simulink model "flightControlSystem"  (R2024b)
settings: Solver=ode3  StartTime=0  StopTime=TFinal  FixedStep=Ts  RelTol=1e-3  EnableMultiTasking=on
undefined symbols (not defined in the file): codertarget, Controller, DiscIntNeverNeededParam, Discrete, Estimator, g, gray, init, Sensors, Time, Ts, var_acc_angle_N, var_bias_gyr_N, var_gyro_p_N, Vehicle
libraries: simulink x37, slpidlib x4, ctrlSharedLib x4, simulink_extras x3, sharedtransform x3, vrlib x2, parrotlib x1
(part 3 of 3)

== system flightControlSystem/Control System/State Estimator/XY Position Estimator/EstimatorVelocity/Angular velocity compensation for optical flow ==
  note: Optical flow readings are affected by both linear and angular velocity of the drone. We need to subtract the effect of angular velocity before using the flow data
  z_estimate : Inport
  Angular velocity w/o bias : Inport  Port=2
  Abs : Abs  SaturateOnIntegerOverflow=off
  Data Type Conversion : DataTypeConversion  SaturateOnIntegerOverflow=off  RndMeth=Floor
  Demux : Demux  Outputs=2
  Gain1 : Gain  Gain=-1
  Mux : Mux  Inputs=2
  Selector : Selector  InputPortWidth=3  IndexOptions=Index vector (dialog)  Indices=[1 2]  OutputSizes=1
  prod : Product  Inputs=**
  angular velocity correction : Outport
  wires:
  Gain1/1 -> Mux/1
  Mux/1 -> Data Type Conversion/1
  Demux/2 -> Gain1/1
  Data Type Conversion/1 -> angular velocity correction/1
  prod/1 -> Demux/1
  z_estimate/1 -> Abs/1
  Demux/1 -> Mux/2
  Selector/1 -> prod/2
  Abs/1 -> prod/1
  Angular velocity w/o bias/1 -> Selector/1

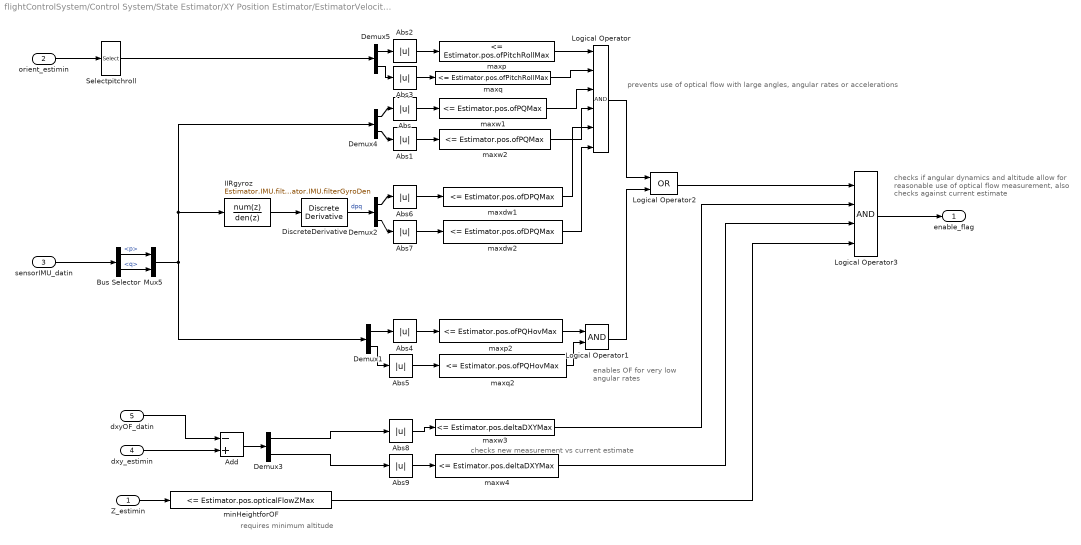
== system flightControlSystem/Control System/State Estimator/XY Position Estimator/EstimatorVelocity/DataHandling ==
  note: prevents use of optical flow with large angles, angular rates or accelerations
  note: enables OF for very
      | low angular rates
  note: checks if angular dynamics and altitude allow for
      | reasonable use of optical flow measurement,
      | also checks against current estimate
  note: checks new measurement vs current estimate
  note: requires minimum altitude
  Z_estimin : Inport
  orient_estimin : Inport  Port=2
  sensorIMU_datin : Inport  Port=3
  dxy_estimin : Inport  Port=4
  dxyOF_datin : Inport  Port=5
  Abs{,1..9} (10 alike) : Abs  SaturateOnIntegerOverflow=off
  Add : Sum  Inputs=-+
  Bus Selector : BusSelector  OutputSignals=p,q
  Demux{1..5} (5 alike) : Demux  Outputs=2
  DiscreteDerivative : simulink/Discrete/Discrete Derivative  gainval=1.0  ICPrevScaledInput=0.0  OutMin=[]  OutMax=[]  OutDataType=fixdt(1, 16)  OutScaling=2^-10  DoSatur=off
  IIRgyroz : DiscreteFilter  Numerator=Estimator.IMU.filterGyroNum  Denominator=Estimator.IMU.filterGyroDen
  Logical Operator : Logic  Inputs=6  AllPortsSameDT=off  OutDataTypeStr=boolean
  Logical Operator1 : Logic  AllPortsSameDT=off  OutDataTypeStr=boolean
  Logical Operator2 : Logic  Operator=OR  AllPortsSameDT=off  OutDataTypeStr=boolean
  Logical Operator3 : Logic  Inputs=4  AllPortsSameDT=off  OutDataTypeStr=boolean
  Mux5 : Mux  Inputs=2
  Selectpitchroll : Selector  InputPortWidth=3  IndexOptions=Index vector (dialog)  Indices=[2 3]  OutputSizes=1
  maxdw1 : simulink/Logic and Bit Operations/Compare To Constant  relop=<=  const=Estimator.pos.ofDPQMax  OutDataTypeStr=boolean
  maxdw2 : simulink/Logic and Bit Operations/Compare To Constant  relop=<=  const=Estimator.pos.ofDPQMax  OutDataTypeStr=boolean
  maxp : simulink/Logic and Bit Operations/Compare To Constant  relop=<=  const=Estimator.pos.ofPitchRollMax  OutDataTypeStr=boolean
  maxp2 : simulink/Logic and Bit Operations/Compare To Constant  relop=<=  const=Estimator.pos.ofPQHovMax  OutDataTypeStr=boolean
  maxq : simulink/Logic and Bit Operations/Compare To Constant  relop=<=  const=Estimator.pos.ofPitchRollMax  OutDataTypeStr=boolean
  maxq2 : simulink/Logic and Bit Operations/Compare To Constant  relop=<=  const=Estimator.pos.ofPQHovMax  OutDataTypeStr=boolean
  maxw1 : simulink/Logic and Bit Operations/Compare To Constant  relop=<=  const=Estimator.pos.ofPQMax  OutDataTypeStr=boolean
  maxw2 : simulink/Logic and Bit Operations/Compare To Constant  relop=<=  const=Estimator.pos.ofPQMax  OutDataTypeStr=boolean
  maxw3 : simulink/Logic and Bit Operations/Compare To Constant  relop=<=  const=Estimator.pos.deltaDXYMax  OutDataTypeStr=boolean
  maxw4 : simulink/Logic and Bit Operations/Compare To Constant  relop=<=  const=Estimator.pos.deltaDXYMax  OutDataTypeStr=boolean
  minHeightforOF : simulink/Logic and Bit Operations/Compare To Constant  relop=<=  const=Estimator.pos.opticalFlowZMax  OutDataTypeStr=boolean
  enable_flag : Outport  VectorParamsAs1DForOutWhenUnconnected=off
  wires:
  minHeightforOF/1 -> Logical Operator3/4
  IIRgyroz/1 -> DiscreteDerivative/1
  Mux5/1 -> Demux1/1, Demux4/1, IIRgyroz/1
  maxw4/1 -> Logical Operator3/3
  maxw3/1 -> Logical Operator3/2
  dxyOF_datin/1 -> Add/1
  Demux3/2 -> Abs9/1
  Demux3/1 -> Abs8/1
  dxy_estimin/1 -> Add/2
  Add/1 -> Demux3/1
  Abs9/1 -> maxw4/1
  Abs8/1 -> maxw3/1
  Logical Operator2/1 -> Logical Operator3/1
  Logical Operator3/1 -> enable_flag/1
  DiscreteDerivative/1 -> Demux2/1  "dpq"
  Demux2/2 -> Abs7/1
  Demux2/1 -> Abs6/1
  Abs7/1 -> maxdw2/1
  Abs6/1 -> maxdw1/1
  Logical Operator1/1 -> Logical Operator2/2
  Demux1/2 -> Abs5/1
  Demux1/1 -> Abs4/1
  Abs5/1 -> maxq2/1
  Abs4/1 -> maxp2/1
  Abs3/1 -> maxq/1
  Abs2/1 -> maxp/1
  Demux4/2 -> Abs1/1
  Demux4/1 -> Abs/1
  Abs1/1 -> maxw2/1
  Abs/1 -> maxw1/1
  Z_estimin/1 -> minHeightforOF/1
  Logical Operator/1 -> Logical Operator2/1
  maxw1/1 -> Logical Operator/3
  Bus Selector/1 -> Mux5/1  "<p>"
  Selectpitchroll/1 -> Demux5/1
  sensorIMU_datin/1 -> Bus Selector/1
  maxq2/1 -> Logical Operator1/2
  Bus Selector/2 -> Mux5/2  "<q>"
  maxp/1 -> Logical Operator/1
  maxw2/1 -> Logical Operator/4
  orient_estimin/1 -> Selectpitchroll/1
  maxdw1/1 -> Logical Operator/5
  maxdw2/1 -> Logical Operator/6
  maxq/1 -> Logical Operator/2
  Demux5/1 -> Abs2/1
  Demux5/2 -> Abs3/1
  maxp2/1 -> Logical Operator1/1

== system flightControlSystem/Control System/State Estimator/XY Position Estimator/EstimatorVelocity/xy velocity w//o angular velocity compensation ==
  note: Optical flow raw readings are converted to velocity in m/s based on the estimated altitude
  optical_flow : Inport
  z_estimate : Inport  Port=2
  " " : Product  Inputs=**
  Compare To Constant : simulink/Logic and Bit Operations/Compare To Constant  relop=<  const=200*4  OutDataTypeStr=boolean
  Counter Free-Running : simulink/Sources/Counter Free-Running  NumBits=32  tsamp=-1
  Gain : Gain  Gain=-1
  Select dxy : Selector  InputPortWidth=3  IndexOptions=Index vector (dialog)  Indices=[1 2]  OutputSizes=1
  Switch : Switch  Criteria=u2 > Threshold  SaturateOnIntegerOverflow=off  InputSameDT=off
  opticalFlowErrorCorrect : Gain  Gain=1.15
  optical_flow_dx_dy : Outport
  wires:
  Select dxy/1 -> optical_flow_dx_dy/1  "optical_flow_dx_dy"
  " "/1 -> opticalFlowErrorCorrect/1
  opticalFlowErrorCorrect/1 -> Switch/3
  Gain/1 -> " "/2
  Switch/1 -> Select dxy/1
  Counter Free-Running/1 -> Compare To Constant/1
  Compare To Constant/1 -> Switch/2
  optical_flow/1 -> " "/1, Switch/1
  z_estimate/1 -> Gain/1

== matlab function flightControlSystem/Image Processing System/Deviation Measurement/MATLAB Function2 ==
  data: err input; iae output; valid input; Ts input; reset input
function iae = metricIAE(err, valid, Ts, reset)
% metricIAE
% Discrete Integral of Absolute Error

persistent acc
if isempty(acc)
    acc = single(0);
end

if reset
    acc = single(0);
else
    if valid ~= 0
        acc = acc + abs(single(err)) * single(Ts);
    end
end

iae = acc;
end

== matlab function flightControlSystem/Image Processing System/Deviation Measurement/MATLAB Function3 ==
  data: err input; itae output; valid input; Ts input; reset input
function itae = metricITAE(err, valid, Ts, reset)
% metricITAE
% Discrete Integral of Time-weighted Absolute Error

persistent acc tNow
if isempty(acc)
    acc  = single(0);
    tNow = single(0);
end

if reset
    acc  = single(0);
    tNow = single(0);
else
    if valid ~= 0
        acc = acc + tNow * abs(single(err)) * single(Ts);
    end
    tNow = tNow + single(Ts);
end

itae = acc;
end

== matlab function flightControlSystem/Image Processing System/Deviation Measurement/MATLAB Function4 ==
  data: R input; G input; B input; d_cm output; e_px output; cm_per_px output; trackW_px output; valid output; offTrack output; IAE output; ITAE output; MAE output; maxErr output; offTime output; offRatio output; validRatio output; debugImg output; headingVec input
function [d_cm, e_px, cm_per_px, trackW_px, valid, offTrack, ...
          IAE, ITAE, MAE, maxErr, offTime, offRatio, validRatio, ...
          debugImg] = fcn(R, G, B, headingVec)

%#codegen

% ============================================================
% PARAMETERS
% ============================================================
rows       = int32(120);
cols       = int32(160);

centerRow  = single(60);
centerCol  = single(80);

redThr     = single(200);   % red detection threshold
trackW_cm  = single(10);    % real track width [cm]
thr_cm     = single(10);    % off-track threshold [cm]
Ts         = single(0.2);   % actual execution sample time of this block

% Cross-section settings
normalHalf     = int32(35);   % half-length of each cross-section [px]
minRunLen      = int32(3);    % minimum contiguous red samples in a section
numSections    = int32(9);    % number of cross-sections along heading

% Section offsets along heading [px]
secOffsets = int32([-12 -9 -6 -3 0 3 6 9 12]);

% ============================================================
% PERSISTENT STATES
% ============================================================
persistent last_d_cm last_e_px last_cm_per_px last_trackW_px
persistent IAE_acc ITAE_acc MAE_sum MAE_count maxErr_val
persistent offTime_acc offCount totalCount validCount tNow
persistent last_trackPtR last_trackPtC
persistent last_hR last_hC
persistent last_dirR last_dirC

if isempty(last_d_cm)
    last_d_cm       = single(0);
    last_e_px       = single(0);
    last_cm_per_px  = single(0);
    last_trackW_px  = single(1);

    IAE_acc         = single(0);
    ITAE_acc        = single(0);
    MAE_sum         = single(0);
    MAE_count       = single(0);
    maxErr_val      = single(0);

    offTime_acc     = single(0);
    offCount        = single(0);
    totalCount      = single(0);
    validCount      = single(0);
    tNow            = single(0);

    last_trackPtR   = centerRow;
    last_trackPtC   = centerCol;

    % Default heading = upward in image plane
    last_hR         = single(-1);
    last_hC         = single(0);

    % Default fitted direction
    last_dirR       = single(-1);
    last_dirC       = single(0);
end

% ============================================================
% HEADING NORMALIZATION
% headingVec is interpreted in image coordinates [row, col]
% ============================================================
hR = single(headingVec(1));
hC = single(headingVec(2));

hNorm = sqrt(hR*hR + hC*hC);

if hNorm > single(1e-6)
    hR = hR / hNorm;
    hC = hC / hNorm;
    last_hR = hR;
    last_hC = hC;
else
    hR = last_hR;
    hC = last_hC;
end

% Normal to heading in image plane
nR = -hC;
nC =  hR;

% ============================================================
% DEBUG IMAGE INIT
% ============================================================
debugImg = zeros(rows, cols, 3, 'uint8');
debugImg(:,:,1) = uint8(R);
debugImg(:,:,2) = uint8(G);
debugImg(:,:,3) = uint8(B);

% ============================================================
% STORAGE FOR VALID CROSS-SECTIONS
% ============================================================
secValid   = false(1, numSections);
secCenterT = zeros(1, numSections, 'single');  % lateral center along normal
secWidth   = zeros(1, numSections, 'single');  % width in px along normal
secPtR     = zeros(1, numSections, 'single');  % detected center point row
secPtC     = zeros(1, numSections, 'single');  % detected center point col
secWeight  = zeros(1, numSections, 'single');

% ============================================================
% SCAN MULTIPLE CROSS-SECTIONS ORTHOGONAL TO HEADING
% ============================================================
for i = 1:numSections
    s = single(secOffsets(i));  % offset along heading from image center

    % Base point of the current cross-section
    baseR = centerRow + s * hR;
    baseC = centerCol + s * hC;

    % Search along normal direction
    currStart = int32(0);
    currLen   = int32(0);
    bestStart = int32(0);
    bestEnd   = int32(-1);
    bestLen   = int32(0);

    prevIsRed = false;

    for t = -normalHalf:normalHalf
        rr = int32(round(baseR + single(t) * nR));
        cc = int32(round(baseC + single(t) * nC));

        isRed = false;

        if rr >= 1 && rr <= rows && cc >= 1 && cc <= cols
            Rv = single(R(rr, cc));
            Gv = single(G(rr, cc));
            Bv = single(B(rr, cc));

            isRed = (Rv - single(0.5)*Gv - single(0.5)*Bv) > redThr;
        end

        if isRed
            if ~prevIsRed
                currStart = t;
                currLen   = int32(1);
            else
                currLen = currLen + int32(1);
            end
        else
            if prevIsRed
                if currLen > bestLen
                    bestLen   = currLen;
                    bestStart = currStart;
                    bestEnd   = t - int32(1);
                end
            end
            currLen = int32(0);
        end

        prevIsRed = isRed;
    end

    % Handle run reaching the end
    if prevIsRed
        if currLen > bestLen
            bestLen   = currLen;
            bestStart = currStart;
            bestEnd   = normalHalf;
        end
    end

    % Accept only meaningful runs
    if bestLen >= minRunLen
        centerT = single(bestStart + bestEnd) * single(0.5);
        widthPx = single(bestEnd - bestStart + int32(1));

        ptR = baseR + centerT * nR;
        ptC = baseC + centerT * nC;

        secValid(i)   = true;
        secCenterT(i) = centerT;
        secWidth(i)   = widthPx;
        secPtR(i)     = ptR;
        secPtC(i)     = ptC;

        % Weight:
        % wider run = more confidence
        % closer to center = slightly more weight
        secWeight(i) = widthPx / (single(1) + single(0.08) * abs(s));
    end
end

% ============================================================
% AGGREGATE CROSS-SECTIONS
% ============================================================
sumW      = single(0);
sumT      = single(0);
sumWidth  = single(0);
sumPtR    = single(0);
sumPtC    = single(0);
numValid  = int32(0);

for i = 1:numSections
    if secValid(i)
        w = secWeight(i);

        sumW     = sumW + w;
        sumT     = sumT + w * secCenterT(i);
        sumWidth = sumWidth + w * secWidth(i);
        sumPtR   = sumPtR + w * secPtR(i);
        sumPtC   = sumPtC + w * secPtC(i);
        numValid = numValid + int32(1);
    end
end

if numValid > 0 && sumW > single(1e-6)
    e = sumT / sumW;            % signed lateral error in pixels along normal
    w_px = sumWidth / sumW;     % estimated track width in pixels
    trackPtR = sumPtR / sumW;   % estimated local centerline point
    trackPtC = sumPtC / sumW;

    if w_px < single(1)
        w_px = single(1);
    end

    cmpp = trackW_cm / w_px;
    d = e * cmpp;

    d_cm       = d;
    e_px       = e;
    cm_per_px  = cmpp;
    trackW_px  = w_px;
    valid      = uint8(1);

    last_d_cm      = d_cm;
    last_e_px      = e_px;
    last_cm_per_px = cm_per_px;
    last_trackW_px = trackW_px;

    last_trackPtR  = trackPtR;
    last_trackPtC  = trackPtC;
else
    d_cm       = last_d_cm;
    e_px       = last_e_px;
    cm_per_px  = last_cm_per_px;
    trackW_px  = last_trackW_px;
    valid      = uint8(0);

    trackPtR   = last_trackPtR;
    trackPtC   = last_trackPtC;
end

% ============================================================
% FIT LOCAL CENTERLINE FROM THE YELLOW POINTS
% weighted line fit / principal direction
% ============================================================
if numValid >= int32(2) && sumW > single(1e-6)
    meanR = sumPtR / sumW;
    meanC = sumPtC / sumW;

    Srr = single(0);
    Scc = single(0);
    Src = single(0);

    for i = 1:numSections
        if secValid(i)
            dr = secPtR(i) - meanR;
            dc = secPtC(i) - meanC;
            w  = secWeight(i);

            Srr = Srr + w * dr * dr;
            Scc = Scc + w * dc * dc;
            Src = Src + w * dr * dc;
        end
    end

    theta = single(0.5) * atan2(single(2) * Src, Srr - Scc);

    dirR = cos(theta);
    dirC = sin(theta);

    dirNorm = sqrt(dirR*dirR + dirC*dirC);
    if dirNorm > single(1e-6)
        dirR = dirR / dirNorm;
        dirC = dirC / dirNorm;

        % Keep orientation roughly aligned with heading to avoid sign flips
        if dirR*hR + dirC*hC < single(0)
            dirR = -dirR;
            dirC = -dirC;
        end

        last_dirR = dirR;
        last_dirC = dirC;
    else
        dirR = last_dirR;
        dirC = last_dirC;
    end
else
    dirR = last_dirR;
    dirC = last_dirC;
end

% ============================================================
% OFF TRACK
% ============================================================
if valid ~= 0
    offTrack = uint8(abs(d_cm) > thr_cm);
else
    offTrack = uint8(0);
end

% ============================================================
% METRICS
% ============================================================
totalCount = totalCount + single(1);

if valid ~= 0
    errAbs = abs(d_cm);

    IAE_acc   = IAE_acc  + errAbs * Ts;
    ITAE_acc  = ITAE_acc + tNow * errAbs * Ts;

    MAE_sum   = MAE_sum + errAbs;
    MAE_count = MAE_count + single(1);

    if errAbs > maxErr_val
        maxErr_val = errAbs;
    end

    validCount = validCount + single(1);

    if offTrack ~= 0
        offTime_acc = offTime_acc + Ts;
        offCount    = offCount + single(1);
    end
end

tNow = tNow + Ts;

IAE     = IAE_acc;
ITAE    = ITAE_acc;
maxErr  = maxErr_val;
offTime = offTime_acc;

if MAE_count > single(0)
    MAE = MAE_sum / MAE_count;
else
    MAE = single(0);
end

if validCount > single(0)
    offRatio = offCount / validCount;
else
    offRatio = single(0);
end

if totalCount > single(0)
    validRatio = validCount / totalCount;
else
    validRatio = single(0);
end

% ============================================================
% DEBUG OVERLAY
% ============================================================

% Draw all accepted section center points (yellow)
for i = 1:numSections
    if secValid(i)
        rr = int32(round(secPtR(i)));
        cc = int32(round(secPtC(i)));

        if rr >= 2 && rr <= rows-1 && cc >= 2 && cc <= cols-1
            for r0 = rr-1:rr+1
                for c0 = cc-1:cc+1
                    debugImg(r0,c0,1) = uint8(255);
                    debugImg(r0,c0,2) = uint8(255);
                    debugImg(r0,c0,3) = uint8(0);
                end
            end
        end
    end
end

% 1) Heading through drone center (cyan)
for k = -45:45
    rr = int32(round(centerRow + single(k) * hR));
    cc = int32(round(centerCol + single(k) * hC));

    if rr >= 1 && rr <= rows && cc >= 1 && cc <= cols
        debugImg(rr,cc,1) = uint8(0);
        debugImg(rr,cc,2) = uint8(255);
        debugImg(rr,cc,3) = uint8(255);
    end
end

% 2) Normal through drone center (magenta)
for k = -45:45
    rr = int32(round(centerRow + single(k) * nR));
    cc = int32(round(centerCol + single(k) * nC));

    if rr >= 1 && rr <= rows && cc >= 1 && cc <= cols
        debugImg(rr,cc,1) = uint8(255);
        debugImg(rr,cc,2) = uint8(0);
        debugImg(rr,cc,3) = uint8(255);
    end
end

% 3) Estimated local centerline fitted from yellow points (blue)
for k = -45:45
    rr = int32(round(trackPtR + single(k) * dirR));
    cc = int32(round(trackPtC + single(k) * dirC));

    if rr >= 1 && rr <= rows && cc >= 1 && cc <= cols
        debugImg(rr,cc,1) = uint8(0);
        debugImg(rr,cc,2) = uint8(0);
        debugImg(rr,cc,3) = uint8(255);
    end
end

% 4) Shortest connection from drone center to local centerline point (white)
numSteps = int32(50);
for k = 0:numSteps
    a = single(k) / single(numSteps);

    rr = int32(round((single(1)-a)*centerRow + a*trackPtR));
    cc = int32(round((single(1)-a)*centerCol + a*trackPtC));

    if rr >= 1 && rr <= rows && cc >= 1 && cc <= cols
        debugImg(rr,cc,1) = uint8(255);
        debugImg(rr,cc,2) = uint8(255);
        debugImg(rr,cc,3) = uint8(255);
    end
end

% 5) Drone center point (green square)
cR = int32(round(centerRow));
cC = int32(round(centerCol));
if cR >= 2 && cR <= rows-1 && cC >= 2 && cC <= cols-1
    for rr = cR-1:cR+1
        for cc = cC-1:cC+1
            debugImg(rr,cc,1) = uint8(0);
            debugImg(rr,cc,2) = uint8(255);
            debugImg(rr,cc,3) = uint8(0);
        end
    end
end

% 6) Track point (white square)
tpR = int32(round(trackPtR));
tpC = int32(round(trackPtC));
if tpR >= 2 && tpR <= rows-1 && tpC >= 2 && tpC <= cols-1
    for rr = tpR-1:tpR+1
        for cc = tpC-1:tpC+1
            debugImg(rr,cc,1) = uint8(255);
            debugImg(rr,cc,2) = uint8(255);
            debugImg(rr,cc,3) = uint8(255);
        end
    end
end

== matlab function flightControlSystem/Image Processing System/MATLAB Function ==
  data: R input; BW output; G input; B input
function BW   = createMask(R, G, B)
%createMask  Threshold RGB image using auto-generated code from colorThresholder app.
%  [BW,MASKEDRGBIMAGE] = createMask(RGB) thresholds image RGB using
%  auto-generated code from the colorThresholder app. The colorspace and
%  range for each channel of the colorspace were set within the app. The
%  segmentation mask is returned in BW, and a composite of the mask and
%  original RGB images is returned in maskedRGBImage.

% Auto-generated by colorThresholder app on 04-Mar-2026
%------------------------------------------------------

% Define thresholds for channel 1 based on histogram settings
channel1Min = 151.000;
channel1Max = 255.000;

% Define thresholds for channel 2 based on histogram settings
channel2Min = 0.000;
channel2Max = 151.000;

% Define thresholds for channel 3 based on histogram settings
channel3Min = 0.000;
channel3Max = 150.000;

% Create mask based on chosen histogram thresholds
sliderBW = (R >= channel1Min ) & (R <= channel1Max) & ...
    (G >= channel2Min ) & (G <= channel2Max) & ...
    (B >= channel3Min ) & (B <= channel3Max);
BW = sliderBW;

end

== matlab function flightControlSystem/Control System/Controller/Position Controller/Position error transformation (Earth to Body frame) ==
  data: yaw input; xy_err_earth input; xy_err_body output
function xy_err_body = fcn(yaw,xy_err_earth)

transformation = [cos(yaw), sin(yaw); -sin(yaw),  cos(yaw)];
xy_err_body = transformation * xy_err_earth;


end

== matlab function flightControlSystem/Image Processing System/Deviation Measurement/MATLAB Function1 ==
  data: R input; d_cm output; G input; B input; e_px output; cm_per_px output; trackW_px output; valid output; offTrack output
function [d_cm, e_px, cm_per_px, trackW_px, valid, offTrack] = fcn(R, G, B)

cols       = int32(160);
centerCol  = single(80);
centerRow  = int32(60);
bandHalf   = int32(8);          % ← Bredere bånd: rader 52–68
redThr     = single(200);       % ← Mildere terskel (prøv 180–220 ved behov)
trackW_cm  = single(10);        % Reell stripebredde i cm
thr_cm     = single(10);        % Dommer-terskel for off-track

persistent last_d_cm last_e_px last_cm_per_px last_trackW_px
if isempty(last_d_cm)
    last_d_cm       = single(0);
    last_e_px       = single(0);
    last_cm_per_px  = single(0);
    last_trackW_px  = single(0);
end

rMin = centerRow - bandHalf;
rMax = centerRow + bandHalf;
numRowsInBand = rMax - rMin + 1;

leftCols  = zeros(1, numRowsInBand, 'int32');
rightCols = zeros(1, numRowsInBand, 'int32');
cntRed    = int32(0);
idx       = 0;

for r = rMin:rMax
    rowRed = false(1, cols);
    for c = 1:cols
        Rv = single(R(r, c));
        Gv = single(G(r, c));
        Bv = single(B(r, c));
        isRed = (Rv - (Gv * single(0.5)) - (Bv * single(0.5))) > redThr;
        rowRed(c) = isRed;
        if isRed
            cntRed = cntRed + 1;
        end
    end
    
    if any(rowRed)
        idx = idx + 1;
        leftCols(idx)  = find(rowRed, 1, 'first');
        rightCols(idx) = find(rowRed, 1, 'last');
    end
end

if idx > 0 && cntRed > 0
    validLeft  = leftCols(1:idx);
    validRight = rightCols(1:idx);
    
    leftCol  = median(validLeft);
    rightCol = median(validRight);
    
    w_px = single(rightCol - leftCol + 1);
    if w_px < single(1)
        w_px = single(1);
    end
    
    cmpp = trackW_cm / w_px;
    trackMidCol = (single(leftCol) + single(rightCol)) * single(0.5);
    e = trackMidCol - centerCol;   % i piksler
    d = e * cmpp;                  % i cm
    
    d_cm       = d;
    e_px       = e;
    cm_per_px  = cmpp;
    trackW_px  = w_px;
    valid      = uint8(1);
    
    last_d_cm      = d_cm;
    last_e_px      = e_px;
    last_cm_per_px = cm_per_px;
    last_trackW_px = trackW_px;
    
else
    d_cm       = last_d_cm;
    e_px       = last_e_px;
    cm_per_px  = last_cm_per_px;
    trackW_px  = last_trackW_px;
    valid      = uint8(0);
end

offTrack = uint8(abs(d_cm) > thr_cm);

end

== matlab function flightControlSystem/Image Processing System/Pure Pursuit/Lookahead Ring ==
  data: BW input; vecRC output double size=[1 2]; headingVec input; debugImg output
function [vecRC, debugImg] = fcn(BW, headingVec)
persistent refRC prevHeadingAngle

if isempty(prevHeadingAngle)
    prevHeadingAngle = 0;
end
if isempty(refRC)
    refRC = [60 80];
end

% Constants
centerRC = [60 80];
rMin = 40;
rMax = 42;
FOV = 0.7;
refStep = 0.001;
alphaAng = 0.35;

% heading
hv1 = headingVec(1);
hv2 = headingVec(2);
newAngle = atan2(hv2, hv1);
angErr = atan2(sin(newAngle - prevHeadingAngle), cos(newAngle - prevHeadingAngle));
prevHeadingAngle = prevHeadingAngle + alphaAng * angErr;
angF = prevHeadingAngle;

% ref point
dRow = refStep * cos(angF);
dCol = refStep * sin(angF);
refRC(1) = 60 - dRow;
refRC(2) = 80 - dCol;

if ~isfinite(refRC(1)) || ~isfinite(refRC(2))
    refRC = centerRC;
end

% fallback if no line detected
if refRC(1) == 60 && refRC(2) == 80
    rMax = 100;
    rMin = 20;
    FOV = pi;
end

anchorLeft = mod(angF + FOV, 2*pi);
anchorRight = mod(angF - FOV, 2*pi);

debugImg = uint8(255) * ones(120,160,'uint8');
debugImg(60,80) = uint8(0);

rRef = round(refRC(1));
cRef = round(refRC(2));
if rRef >= 1 && rRef <= 120 && cRef >= 1 && cRef <= 160
    debugImg(rRef,cRef) = uint8(0);
end

% Pixel scan
sumVec = [0 0];
redCount = 0;

for c = 1:160
    for r = 1:120
        dR = r - centerRC(1);
        dC = c - centerRC(2);
        rad = sqrt(dR*dR + dC*dC);
        if rad < rMin || rad > rMax
            continue;
        end

        yaw = atan2(dC, dR);
        yaw2 = mod(yaw, 2*pi);

        if anchorLeft < anchorRight
            flag = (yaw2 <= 2*pi && yaw2 >= anchorRight) || ...
                   (yaw2 <= anchorLeft && yaw2 >= 0);
        else
            flag = (yaw2 <= anchorLeft && yaw2 >= anchorRight);
        end

        if ~flag
            continue;
        end

        debugImg(r,c) = uint8(120);

        px = BW(r,c);
        if ~islogical(px)
            hit = (px > 0);
        else
            hit = px;
        end

        if hit
            redCount = redCount + 1;
            sumVec(1) = sumVec(1) + (r - round(refRC(1)));
            sumVec(2) = sumVec(2) + (c - round(refRC(2)));
            debugImg(r,c) = uint8(0);
        end
    end
end

% Average vec
if redCount <= 0
    vecRC = [0 0];
else
    vecRC = sumVec / redCount;
    if ~isfinite(vecRC(1)) || ~isfinite(vecRC(2))
        vecRC = [0 0];
    end
end
end

== matlab function flightControlSystem/Image Processing System/Pure Pursuit/Close Ring ==
  data: BW input; pixelVecRC output; headingVec input; debugImg output
function [pixelVecRC, debugImg] = fcn(BW, headingVec)
persistent refPointRC prevHeadingAngle coastCounter lastPixelVecRC

% Constants
rMin = 20;
rMax = 24;
FOV = 1.3;
refStep = 0.001;
alphaAng = 0.2;
eps = 1e-10;

%init
if isempty(prevHeadingAngle)
    prevHeadingAngle = 0;
end
if isempty(refPointRC)
    refPointRC = [60 80];
end
if isempty(coastCounter)
    coastCounter = 0;
end
if isempty(lastPixelVecRC)
    lastPixelVecRC = [0 0];
end
imgCenterRC = [60 80]; % [row, col]

% Heading
newHeadingAngle = atan2(headingVec(2), headingVec(1));
angleDiff = atan2(sin(newHeadingAngle - prevHeadingAngle), cos(newHeadingAngle - prevHeadingAngle));
prevHeadingAngle = prevHeadingAngle + alphaAng * angleDiff;
blendedAngle = prevHeadingAngle;
dRowRef = refStep * cos(blendedAngle);
dColRef = refStep * sin(blendedAngle);
refPointRC(1) = 60 - dRowRef;
refPointRC(2) = 80 - dColRef;
if ~isfinite(refPointRC(1)) || ~isfinite(refPointRC(2))
    refPointRC = [60 80];
end

fallbackActive = (abs(refPointRC(1) - 60) < eps && abs(refPointRC(2) - 80) < eps);
fallbackActive = fallbackActive || (coastCounter >= 5);

% Debug image
debugImg = 255 * ones(120, 160, 'uint8');
refR = round(refPointRC(1));
refC = round(refPointRC(2));
if refR >= 1 && refR <= 120 && refC >= 1 && refC <= 160
    debugImg(refR, refC) = 0;
end
debugImg(60, 80) = 0;

if fallbackActive
    rMax = 100;
    rMin = 20;
    FOV = 3.12;
end

fovLeftEdge = mod((blendedAngle + FOV), 2*pi);
fovRightEdge = mod((blendedAngle - FOV), 2*pi);

% Vectorized processing
[colGrid, rowGrid] = meshgrid(1:160, 1:120);
dRow = rowGrid - imgCenterRC(1);
dCol = colGrid - imgCenterRC(2);
dist = sqrt(dRow.^2 + dCol.^2);
inRange = (dist >= rMin) & (dist <= rMax);
pixelYaw = atan2(dCol, dRow);
pixelYaw2 = mod(pixelYaw, 2*pi);
if fovLeftEdge < fovRightEdge
    inFOV = (pixelYaw2 >= fovRightEdge) | (pixelYaw2 <= fovLeftEdge);
else
    inFOV = (pixelYaw2 <= fovLeftEdge) & (pixelYaw2 >= fovRightEdge);
end
turnDiff = angleDiff;
if abs(turnDiff) > deg2rad(15)
    relYawRaw = pixelYaw - blendedAngle;
    relYaw = atan2(sin(relYawRaw), cos(relYawRaw));
    turnDir = sign(turnDiff);
    inTurn = (turnDir .* relYaw >= 0);
else
    inTurn = true(size(pixelYaw));
end
dotProd = dRow .* cos(blendedAngle) + dCol .* sin(blendedAngle);
inFront = dotProd >= 0;

if fallbackActive
    inFront = true(size(dotProd));
end

lineMask = BW > 0;
fullMask = inRange & inFOV & inTurn & inFront & lineMask;

% Debug
inDebug = inRange & inFOV & inTurn & inFront;
debugImg(inDebug) = 120;
debugImg(fullMask) = 0;
whiteCount = nnz(fullMask);

if whiteCount > 0
    sumRow = sum(rowGrid(fullMask));
    sumCol = sum(colGrid(fullMask));
    sumPixelVec = [sumRow - whiteCount * refR, sumCol - whiteCount * refC];
    pixelVecRC = sumPixelVec / whiteCount;
    lastPixelVecRC = pixelVecRC;
    coastCounter = 0;
else
    coastCounter = coastCounter + 1;
    if coastCounter <= 15
        pixelVecRC = lastPixelVecRC;
    else
        pixelVecRC = [0 0];
    end
end
if (isnan(pixelVecRC(1)) || isnan(pixelVecRC(2)))
    pixelVecRC = [0 0];
end
end

== matlab function flightControlSystem/Image Processing System/Deviation Measurement/MATLAB Function ==
  data: R input; R_out output; G input; B input; G_out output; B_out output
function [R_out, G_out, B_out] = fcn(R, G, B)

R_out = R;
G_out = G;
B_out = B;

rowC = 60;
colC = 80;
thickness = 1;

for t = -thickness:thickness
    currRow = rowC + t;
    if currRow >= 1 && currRow <= 120
        for cc = colC - 5 : colC + 5
            if cc >= 1 && cc <= 160
                R_out(currRow, cc) = 0;
                G_out(currRow, cc) = 255;
                B_out(currRow, cc) = 0;
            end
        end
    end
end

for t = -thickness:thickness
    currCol = colC + t;
    if currCol >= 1 && currCol <= 160
        for rr = rowC - 5 : rowC + 5
            if rr >= 1 && rr <= 120
                R_out(rr, currCol) = 0;
                G_out(rr, currCol) = 255;
                B_out(rr, currCol) = 0;
            end
        end
    end
end

end

== matlab function flightControlSystem/Image Processing System/Land/CircleDetect ==
  data: BW input; landCmd output; directionRC output; circleDetected output
function [landCmd, directionRC, circleDetected] = fcn(BW)
persistent circleLock blobAnalyzer alignCounter

if isempty(circleLock)
    circleLock = false;
    alignCounter = 0;
end

landCmd = 0;
directionRC = [0 0];
circleDetected = circleLock;
maxArea = 0;
minEcc = 1;
numCircularBlobs = 0;

imgRows = 120;
imgCols = 160;
alignFrames = 3;
minDetectArea = 300;
minLandArea = 1200;
maxECC = 0.5;
minCircular = 0.8; % 4*pi*area/x^2 > 0.8

if isempty(blobAnalyzer)
    blobAnalyzer = vision.BlobAnalysis(...
        'AreaOutputPort', true, ...
        'CentroidOutputPort', true, ...
        'BoundingBoxOutputPort', false, ...
        'EccentricityOutputPort', true, ...
        'PerimeterOutputPort', true, ...
        'MinimumBlobArea', 100, ...
        'MaximumBlobArea', 5000, ...
        'MaximumCount', 50);
end

coder.varsize('areas', [50 1], [1 0]);
coder.varsize('centroids', [50 2], [1 0]);
coder.varsize('eccentricities', [50 1], [1 0]);
coder.varsize('perimeters', [50 1], [1 0]);

if islogical(BW)
    mask = BW;
else
    mask = BW > 0;
end

mask = bwareaopen(mask, 100);
[areas, centroids, eccentricities, perimeters] = blobAnalyzer(mask);
detected = false;
center = [];

if ~isempty(areas) % Calc circularity
    circularities = zeros(size(areas));
    for i = 1:length(areas)
        if perimeters(i) > 0
            circularities(i) = 4 * pi * double(areas(i)) / (double(perimeters(i))^2);
        end
    end

    % Filter - low ecc, high circularity, sufficient area
    circMask = (eccentricities < maxECC) & ...
               (circularities > minCircular) & ...
               (areas >= minDetectArea);

    numCircularBlobs = double(sum(circMask));

    if numCircularBlobs > 0
        circAreas = areas(circMask);
        circEcc   = eccentricities(circMask);

        [tempMax, relIdx] = max(circAreas);
        maxArea = double(tempMax);
        minEcc  = min(circEcc);

        idxList = find(circMask);
        if ~isempty(idxList) && relIdx <= length(idxList)
            idx = idxList(relIdx);
            center = centroids(idx, :);
            directionRC = [center(2) - 60, center(1) - 80];
            detected = true;

            if center(1) > 70 && center(1) < 90 && center(2) > 50 && center(2) < 70
                alignCounter = alignCounter + 1;
                if alignCounter >= alignFrames && tempMax > minLandArea
                    landCmd = 1;
                end
            else
                alignCounter = 0;
            end
        else
            alignCounter = 0;
        end
    else
        alignCounter = 0;
    end
else
    alignCounter = 0;
end

% Lock
if ~circleLock
    if detected
        circleLock = true;
    end
else
    if ~detected
        circleLock = false;
        alignCounter = 0;
    end
end

circleDetected = circleLock;

end

== stateflow chart flightControlSystem/Control System/Path Planning/Chart ==
  state Hover
    entry:
    pos_ref = [xEst; yEst; -1.0];
  state Follow
    entry:
    yin_f  = 0;
    alpha  = 0.85;
    yDead  = 0.00003;
    yMax   = 0.002;
    during:
    % Lat filter
    yin_f = (1 - alpha)*yin_f + alpha*yIN;
    if (yin_f < yDead && yin_f > -yDead)
    yin_f = 0;
    end
    % sat
    if (yin_f >  yMax) yin_f =  yMax; end
    if (yin_f < -yMax) yin_f = -yMax; end
    % ref
    pos_ref(1) = pos_ref(1) + xIN;
    pos_ref(2) = pos_ref(2) + yin_f;
    pos_ref(3) = -1.0;
  state Land
    during:
    pos_ref(3) = (pos_ref(3) + 0.2*(0.05 - pos_ref(3)))-0.025;
    %if (abs(xEst) < 0.1 && abs(yEst) < 0.1)
    %else
    % pos_ref(1) = xEst;
    % pos_ref(2) = yEst;
    %end
  state hardLand
    entry:
    pos_ref(3) = 0.0;
  (default) -> Hover
  Hover -> Follow : [after(0.65,sec)]
  Follow -> Land : [circleDetect == 1]
  Land -> hardLand : after(2, sec)
  data: xEst input; yEst input; xIN input; yIN input; circleDetect input; pos_ref output; yMax local; alpha local; yin_f local; yDead local
